simulink model "SISO_3D"  (R2022a)
settings: Solver=VariableStepAuto  StartTime=0.0  StopTime=1  RelTol=1e-3
values from neighbouring files (symbols this model uses):
  d0 = 1e-09    [system_parameters.mat]    (also in system_parameters_3d.mat)
  fs = 30000    [system_parameters.mat]    (also in system_parameters_3d.mat = 20000)
  g = 0.0011    [system_parameters.mat]    (also in system_parameters_3d.mat)
  Ga = 1.2e-09    [system_parameters.mat]
  Gax = 2.35e-07    [system_parameters_3d.mat]
  Gc = 1000000000    [system_parameters.mat]    (also in system_parameters_3d.mat)
  Gcc = 0.03    [system_parameters_3d.mat]
  Gcs = 200    [system_parameters_3d.mat]
  Gv = 15    [system_parameters.mat]    (also in system_parameters_3d.mat)
  k = 2.29    [hinf_design.m]    (also in system_parameters.mat = 16500000000; system_parameters_3d.mat = 16500000000)
  R = conv(Rp,Hr)    [bezoutd_AB.m]    (also in hinf_design.m = [ctrl_Hinfd_n]; trans_sens_funct.m = tf(R, 1, Te, 'Variable', 'z^-1'))
  S = conv(Sp,Hs)    [bezoutd_AB.m]    (also in hinf_design.m = [ctrl_Hinfd_d]; mean_var.m = load(fig, '-mat'); trans_sens_funct.m = tf(S, 1, Te, 'Variable', 'z^-1'))
  vb = 1.025    [system_parameters.mat]    (also in system_parameters_3d.mat)
  wa = 120000    [hinf_design.m]    (also in system_parameters.mat)
  wax = 630    [system_parameters_3d.mat]
  wc = 13000    [system_parameters.mat]    (also in system_parameters_3d.mat)
  wcc = 100    [system_parameters_3d.mat]
  wcs = 8500    [system_parameters_3d.mat]
  wv = 4000    [hinf_design.m]    (also in system_parameters.mat; system_parameters_3d.mat)
  zeta = 0.9    [system_parameters.mat]
  zetax = 0.5    [system_parameters_3d.mat]
libraries: simulink x2, slpidlib x1, spsTriangleGeneratorLib x1
settings Model: Creator=doamarar  LastModifiedBy=doamarar
settings DataIOCC: InspectSignalLogs=on  ReturnWorkspaceOutputs=off

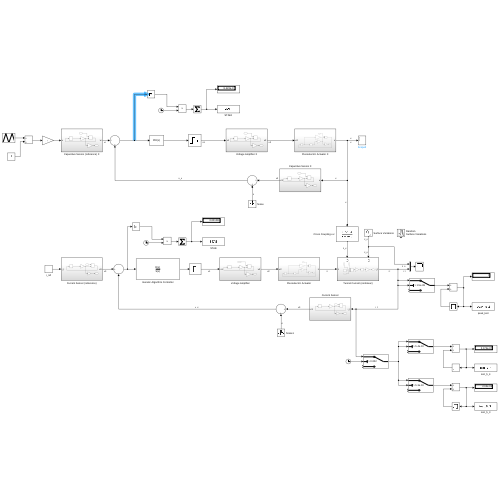
[thumbnail: Simulink's stored preview of the top-level diagram]
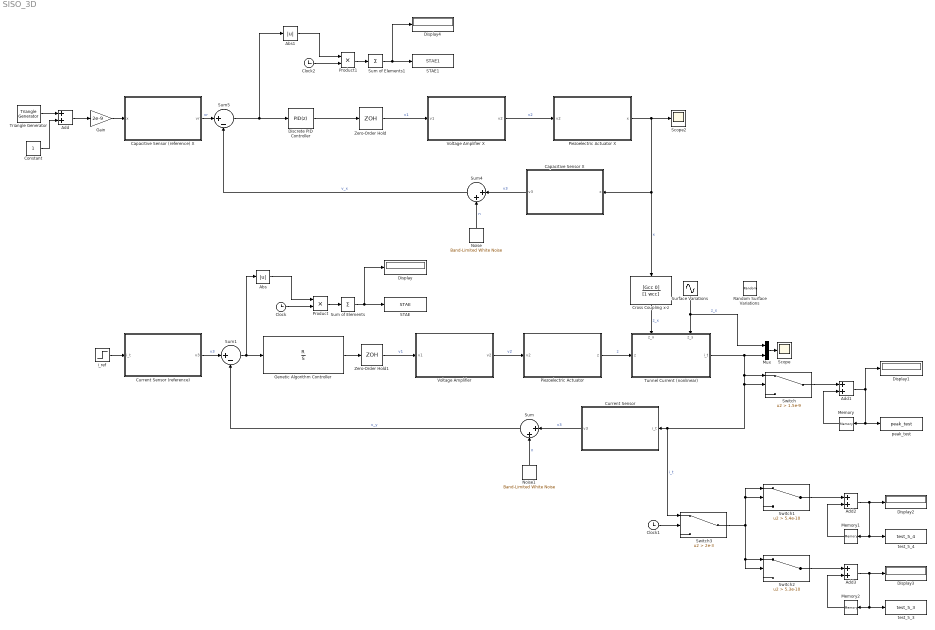
== system SISO_3D ==
  Abs : Abs  SaturateOnIntegerOverflow=off
  Abs1 : Abs  SaturateOnIntegerOverflow=off
  Add{,1..3} (4 alike) : Sum
  Capacitive Sensor (reference) X : Subsystem
  Capacitive Sensor X : Subsystem
  Clock : Clock
  Clock1 : Clock
  Clock2 : Clock
  Constant : Constant
  Cross Coupling x-z : TransferFcn  Numerator=[Gcc 0]  Denominator=[1 wcc]
  Current Sensor : Subsystem
  Current Sensor (reference) : Subsystem
  Discrete PID Controller : slpidlib/PID Controller  Controller=PID  Form=Parallel  TimeDomain=Discrete-time  UseExternalTs=off  SampleTime=5e-5  IntegratorMethod=Forward Euler  FilterMethod=Forward Euler  ControllerParametersSource=internal  P=1082.19714511777  I=465103.622989664  UseKiTs=off  D=0.357644807463686  N=24065.7112678099  UseFilter=on  TunerSelectOption=Transfer Function Based (PID Tuner App)  InitialConditionSource=internal  InitialConditionForIntegrator=0  InitialConditionForFilter=0  DifferentiatorICPrevScaledInput=0  ExternalReset=none  TrackingMode=off  Kt=1  LimitOutput=off  SatLimitsSource=internal  UpperSaturationLimit=inf  LowerSaturationLimit=-inf  LinearizeAsGain=off  AntiWindupMode=none  Kb=1  POutMin=[]  POutMax=[]  IOutMin=[]  IOutMax=[]  DOutMin=[]  DOutMax=[]  NOutMin=[]  NOutMax=[]  SumOutMin=[]  SumOutMax=[]  SaturationOutMin=[]  SaturationOutMax=[]  PParamMin=[]  PParamMax=[]  IParamMin=[]  IParamMax=[]  DParamMin=[]  DParamMax=[]  NParamMin=[]  NParamMax=[]  KbParamMin=[]  KbParamMax=[]  KtParamMin=[]  KtParamMax=[]  KbOutMin=[]  KbOutMax=[]  KtOutMin=[]  KtOutMax=[]  IntegratorOutMin=[]  IntegratorOutMax=[]  FilterOutMin=[]  FilterOutMax=[]  SumI1OutMin=[]  SumI1OutMax=[]  SumI2OutMin=[]  SumI2OutMax=[]  SumI3OutMin=[]  SumI3OutMax=[]  SumI4OutMin=[]  SumI4OutMax=[]  SumDOutMin=[]  SumDOutMax=[]  DifferentiatorOutMin=[]  DifferentiatorOutMax=[]  FilterDiffOutCoefMin=[]  FilterDiffOutCoefMax=[]  ReciprocalOutMin=[]  ReciprocalOutMax=[]  SumDenOutMin=[]  SumDenOutMax=[]  SumNumOutMin=[]  SumNumOutMax=[]  DivideOutMin=[]  DivideOutMax=[]  UdiffTsProdOutMin=[]  UdiffTsProdOutMax=[]  NTsProdOutMin=[]  NTsProdOutMax=[]  UintegralTsProdOutMin=[]  UintegralTsProdOutMax=[]  UngainTsProdOutMin=[]  UngainTsProdOutMax=[]  IntegratorContinuousStateAttributes=''  IntegratorStateMustResolveToSignalObject=off  IntegratorRTWStateStorageClass=Auto  FilterContinuousStateAttributes=''  FilterStateMustResolveToSignalObject=off  FilterRTWStateStorageClass=Auto  ParallelPVariant=InternalParameters  IdealPVariant=Disabled  IVariant=InternalParameters  DVariant=InternalParameters  IntegratorVariant=Discrete  SatVariant=Disabled  AWVariant=Passthrough  PCopyVariant=Disabled  TRVariant=Disabled  FdbkBlocksVariant=Forward  IdealPFdbkVariant=Disabled  SatFdbkVariant=Disabled  DerivativeFilterVariant=ForwardEulerFilter  NVariant=InternalParameters  NCopyVariant=Disabled  FilterICVariant=InternalICsFilter  IntegratorICVariant=InternalICs  ExternalResetVariant=Disabled  TRSumVariant=Passthrough  SumFdbkVariant=Disabled  SumVariant=Sum_PID  TsampFilterVariant=InternalTs  TsampNgainVariant=Passthrough  TsampIntegralVariant=Passthrough  ExternalSaturationOutDataTypeStr=Inherit: Same as second input  aMode=0
  Display{,1..4} (5 alike) : Display
  Gain : Gain  Gain=2e-9
  Genetic Algorithm Controller : DiscreteFilter  Numerator=R  Denominator=S  SampleTime=1/fs
  Memory : Memory
  Memory1 : Memory
  Memory2 : Memory
  Mux : Mux  Inputs=2
  Noise : simulink/Sources/Band-Limited White Noise  Cov=[0.00000000000000001]  Ts=5e-5  seed=[23341]
  Noise1 : simulink/Sources/Band-Limited White Noise  Cov=[0.000000001]  Ts=1/fs  seed=[23341]
  Piezoelectric Actuator : Subsystem
  Piezoelectric Actuator X : Subsystem
  Product : Product
  Product1 : Product
  Random Surface Variations : RandomNumber  Variance=2*10^-25  SampleTime=0.0000333333
  STAE : ToWorkspace  VariableName=STAE  SampleTime=-1
  STAE1 : ToWorkspace  VariableName=STAE1  SampleTime=-1
  Scope : Scope
  Scope2 : Scope
  Sum : Sum  Inputs=|++
  Sum of Elements : Sum  Inputs=+
  Sum of Elements1 : Sum  Inputs=+
  Sum1 : Sum  Inputs=|+-
  Sum4 : Sum  Inputs=|++
  Sum5 : Sum  Inputs=|+-
  Surface Variations : Sin  Amplitude=5*10^-11  Frequency=800  SampleTime=1/fs
  Switch : Switch  Criteria=u2 > Threshold  Threshold=1.5e-9  SaturateOnIntegerOverflow=off  InputSameDT=off
  Switch1 : Switch  Criteria=u2 > Threshold  Threshold=5.4e-10  SaturateOnIntegerOverflow=off  InputSameDT=off
  Switch2 : Switch  Criteria=u2 > Threshold  Threshold=5.3e-10  SaturateOnIntegerOverflow=off  InputSameDT=off
  Switch3 : Switch  Criteria=u2 > Threshold  Threshold=2e-3  SaturateOnIntegerOverflow=off  InputSameDT=off
  Triangle Generator : spsTriangleGeneratorLib/Triangle Generator  Freq=20  Phase=0  Ts=5e-5
  Tunnel Current (nonlinear) : Subsystem
      settings: PortSchema="{\"entries\":[{\"content\":{\"sides\":[{\"content\":{\"connectorIds\":[\"In1\"]},\"type\":\"ConnectorPlacement.EquallySpacedRectSide\",\"uuid\":\"147d123d-45a5-4220-b41f-835da98fb0cd\"},{\"content\":{\"connectorIds\":[\"Out1\"],\"side\":\"RIGHT\"},\"type\":\"ConnectorPlacement.EquallySpacedRectSide\",\"uuid\":\"1a05abba-b8fc-4d61-92c8-15761dd3dd6b\"},{\"content\":{\"connectorIds\":[\"In2\",\"In3\"],\"side\":\"TOP\"},\"type\":\"ConnectorPlacement.EquallySpacedRectSide\",\"uuid\":\"bc9d4ee1-4dd7-4150-9ece-b291902d4347\"}]},\"type\":\"ConnectorPlacement.EquallySpacedConnector\",\"uuid\":\"916abd9f-079e-4be3-a864-fdb35439c6f4\"}],\"packageUris\":[\"http://schema.mathworks.com/mf0/Connector/R2020b\"],\"version\":\"1.0\"}"
  Voltage Amplifier : Subsystem
  Voltage Amplifier X : Subsystem
  Zero-Order Hold : ZeroOrderHold  SampleTime=5e-5
  Zero-Order Hold1 : ZeroOrderHold  SampleTime=1/fs
  i_ref : Step  Time=0  After=0.5*10^-9  SampleTime=1/fs
  peak_test : ToWorkspace  VariableName=peak_test  SampleTime=-1
  test_5_3 : ToWorkspace  VariableName=test_5_3  SampleTime=-1
  test_5_4 : ToWorkspace  VariableName=test_5_4  SampleTime=-1
  wires:
  Capacitive Sensor (reference) X/1(vr) -> Sum5/1  "vr"
  Noise/1 -> Sum4/2  "n"
  Discrete PID Controller/1 -> Zero-Order Hold/1
  Sum4/1 -> Sum5/2  "v_x"
  Triangle Generator/1 -> Add/1
  Add/1 -> Gain/1
  Constant/1 -> Add/2
  Capacitive Sensor X/1(v3) -> Sum4/1  "v3"
  Piezoelectric Actuator X/1(x) -> Scope2/1, Cross Coupling x-z/1, Capacitive Sensor X/1(x)  "x"
  Voltage Amplifier X/1(v2) -> Piezoelectric Actuator X/1(v2)  "v2"
  Gain/1 -> Capacitive Sensor (reference) X/1(x)
  Zero-Order Hold/1 -> Voltage Amplifier X/1(v1)  "v1"
  Sum/1 -> Sum1/2  "v_y"
  Current Sensor/1(v3) -> Sum/1  "v3"
  Add1/1 -> Memory/1, peak_test/1, Display1/1
  Zero-Order Hold1/1 -> Voltage Amplifier/1(v1)  "v1"
  Memory2/1 -> Add3/2
  Add2/1 -> Display2/1, test_5_4/1, Memory1/1
  Sum of Elements/1 -> Display/1, STAE/1
  Switch2/1 -> Add3/1
  i_ref/1 -> Current Sensor (reference)/1(i_t)
  Genetic Algorithm Controller/1 -> Zero-Order Hold1/1
  Voltage Amplifier/1(v2) -> Piezoelectric Actuator/1(v2)  "v2"
  Noise1/1 -> Sum/2  "n"
  Memory/1 -> Add1/2
  Surface Variations/1 -> Mux/1, Tunnel Current (nonlinear)/3(z_s)  "z_s"
  Switch1/1 -> Add2/1
  Sum1/1 -> Genetic Algorithm Controller/1, Abs/1
  Mux/1 -> Scope/1
  Memory1/1 -> Add2/2
  Tunnel Current (nonlinear)/1(i_t) -> Mux/2, Switch3/1, Current Sensor/1(i_t), Switch/2, Switch/1  "i_t"
  Clock/1 -> Product/2
  Add3/1 -> Display3/1, test_5_3/1, Memory2/1
  Current Sensor (reference)/1(v3) -> Sum1/1  "v3"
  Clock1/1 -> Switch3/2
  Switch/1 -> Add1/1
  Switch3/1 -> Switch2/2, Switch2/1, Switch1/2, Switch1/1
  Piezoelectric Actuator/1(z) -> Tunnel Current (nonlinear)/1(z)  "z"
  Product/1 -> Sum of Elements/1
  Abs/1 -> Product/1
  Cross Coupling x-z/1 -> Tunnel Current (nonlinear)/2(z_x)  "z_x"
  Product1/1 -> Sum of Elements1/1
  Sum5/1 -> Abs1/1, Discrete PID Controller/1
  Abs1/1 -> Product1/1
  Sum of Elements1/1 -> Display4/1, STAE1/1
  Clock2/1 -> Product1/2

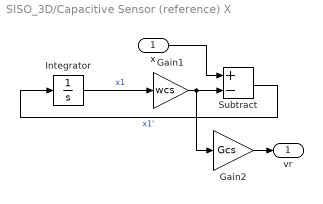
== system SISO_3D/Capacitive Sensor (reference) X ==
  x : Inport
  Gain1 : Gain  Gain=wcs
  Gain2 : Gain  Gain=Gcs
  Integrator : Integrator
  Subtract : Sum  Inputs=+-
  vr : Outport
  wires:
  x/1 -> Subtract/1
  Gain2/1 -> vr/1
  Gain1/1 -> Subtract/2, Gain2/1
  Subtract/1 -> Integrator/1  "x1'"
  Integrator/1 -> Gain1/1  "x1"

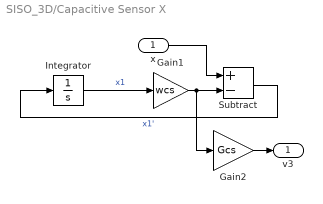
== system SISO_3D/Capacitive Sensor X ==
  x : Inport
  Gain1 : Gain  Gain=wcs
  Gain2 : Gain  Gain=Gcs
  Integrator : Integrator
  Subtract : Sum  Inputs=+-
  v3 : Outport
  wires:
  x/1 -> Subtract/1
  Gain2/1 -> v3/1
  Gain1/1 -> Subtract/2, Gain2/1
  Subtract/1 -> Integrator/1  "x1'"
  Integrator/1 -> Gain1/1  "x1"

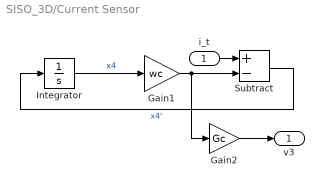
== system SISO_3D/Current Sensor ==
  i_t : Inport
  Gain1 : Gain  Gain=wc
  Gain2 : Gain  Gain=Gc
  Integrator : Integrator
  Subtract : Sum  Inputs=+-
  v3 : Outport
  wires:
  Gain2/1 -> v3/1
  Integrator/1 -> Gain1/1  "x4"
  Gain1/1 -> Gain2/1, Subtract/2
  i_t/1 -> Subtract/1
  Subtract/1 -> Integrator/1  "x4'"

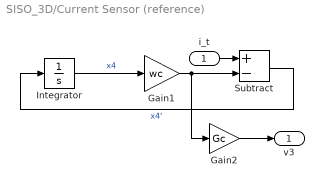
== system SISO_3D/Current Sensor (reference) ==
  i_t : Inport
  Gain1 : Gain  Gain=wc
  Gain2 : Gain  Gain=Gc
  Integrator : Integrator
  Subtract : Sum  Inputs=+-
  v3 : Outport
  wires:
  Gain2/1 -> v3/1
  Integrator/1 -> Gain1/1  "x4"
  Gain1/1 -> Gain2/1, Subtract/2
  i_t/1 -> Subtract/1
  Subtract/1 -> Integrator/1  "x4'"

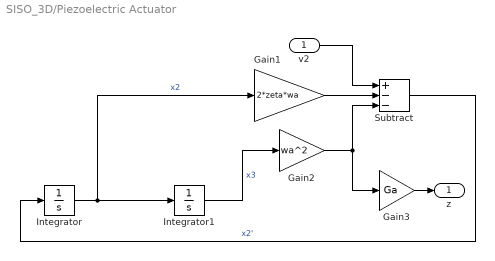
== system SISO_3D/Piezoelectric Actuator ==
  v2 : Inport
  Gain1 : Gain  Gain=2*zeta*wa
  Gain2 : Gain  Gain=wa^2
  Gain3 : Gain  Gain=Ga
  Integrator : Integrator
  Integrator1 : Integrator
  Subtract : Sum  Inputs=+--
  z : Outport
  wires:
  Subtract/1 -> Integrator/1  "x2'"
  Gain1/1 -> Subtract/2
  v2/1 -> Subtract/1
  Gain2/1 -> Gain3/1, Subtract/3
  Integrator/1 -> Gain1/1, Integrator1/1  "x2"
  Gain3/1 -> z/1
  Integrator1/1 -> Gain2/1  "x3"

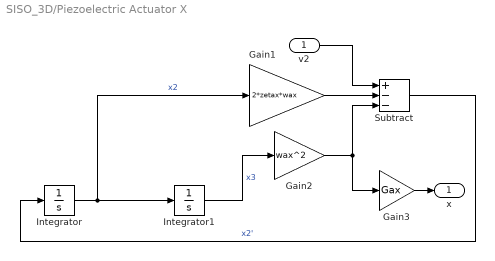
== system SISO_3D/Piezoelectric Actuator X ==
  v2 : Inport
  Gain1 : Gain  Gain=2*zetax*wax
  Gain2 : Gain  Gain=wax^2
  Gain3 : Gain  Gain=Gax
  Integrator : Integrator
  Integrator1 : Integrator
  Subtract : Sum  Inputs=+--
  x : Outport
  wires:
  Integrator1/1 -> Gain2/1  "x3"
  Gain3/1 -> x/1
  Integrator/1 -> Integrator1/1, Gain1/1  "x2"
  Gain2/1 -> Gain3/1, Subtract/3
  v2/1 -> Subtract/1
  Gain1/1 -> Subtract/2
  Subtract/1 -> Integrator/1  "x2'"

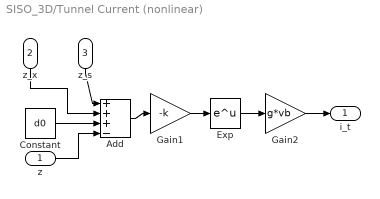
== system SISO_3D/Tunnel Current (nonlinear) ==
  z : Inport
  z_x : Inport  Port=2
  z_s : Inport  Port=3
  Add : Sum  Inputs=+++-
  Constant : Constant  Value=d0
  Exp : Math
  Gain1 : Gain  Gain=-k
  Gain2 : Gain  Gain=g*vb
  i_t : Outport
  wires:
  Add/1 -> Gain1/1
  Gain1/1 -> Exp/1
  Exp/1 -> Gain2/1
  Gain2/1 -> i_t/1
  z/1 -> Add/4
  Constant/1 -> Add/3
  z_s/1 -> Add/1
  z_x/1 -> Add/2

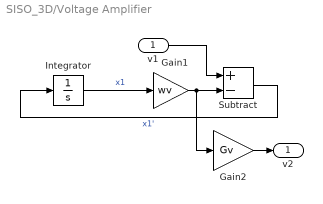
== system SISO_3D/Voltage Amplifier ==
  v1 : Inport
  Gain1 : Gain  Gain=wv
  Gain2 : Gain  Gain=Gv
  Integrator : Integrator
  Subtract : Sum  Inputs=+-
  v2 : Outport
  wires:
  Integrator/1 -> Gain1/1  "x1"
  Subtract/1 -> Integrator/1  "x1'"
  Gain1/1 -> Gain2/1, Subtract/2
  Gain2/1 -> v2/1
  v1/1 -> Subtract/1

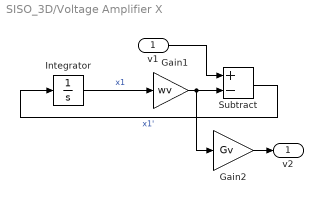
== system SISO_3D/Voltage Amplifier X ==
  v1 : Inport
  Gain1 : Gain  Gain=wv
  Gain2 : Gain  Gain=Gv
  Integrator : Integrator
  Subtract : Sum  Inputs=+-
  v2 : Outport
  wires:
  v1/1 -> Subtract/1
  Gain2/1 -> v2/1
  Gain1/1 -> Subtract/2, Gain2/1
  Subtract/1 -> Integrator/1  "x1'"
  Integrator/1 -> Gain1/1  "x1"
